simulink model "dr_screening_workflow"  (R2026a)
settings: Solver=FixedStepDiscrete  StopTime=sim_days*86400  FixedStep=fixed_step
values from neighbouring files (symbols this model uses):
  ai_time_s = 1.06    [run_workflow_sim.m]
  bandwidth_Mbps = 5    [run_workflow_sim.m]
  fixed_step = 5    [run_workflow_sim.m]
  image_MB = 0.35    [run_workflow_sim.m]
  images_per_patient = 2    [run_workflow_sim.m]
  n_ai_workers = 2    [run_workflow_sim.m]
  n_cameras = 6    [run_workflow_sim.m]
  n_reviewers = base_nr    (= 2)    [run_workflow_sim.m]
  patients_per_day = annual_volume/365    (= 273.97260274)    [run_workflow_sim.m]
  referral_frac = 0.30    (= 0.3)    [run_workflow_sim.m]
  review_time_s = 120    [run_workflow_sim.m]
  Tdrain = 60    [run_workflow_sim.m]
undefined symbols (not defined in the file or in its folder): DiscIntNeverNeededParam
settings Model: Creator=giridharansrinivasannaidu  LastModifiedBy=giridharansrinivasannaidu

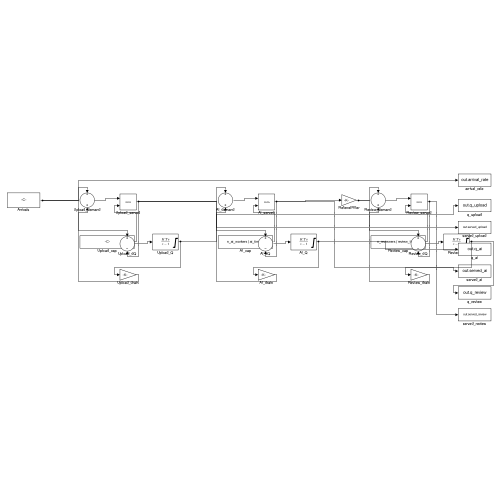
[thumbnail: Simulink's stored preview of the top-level diagram]
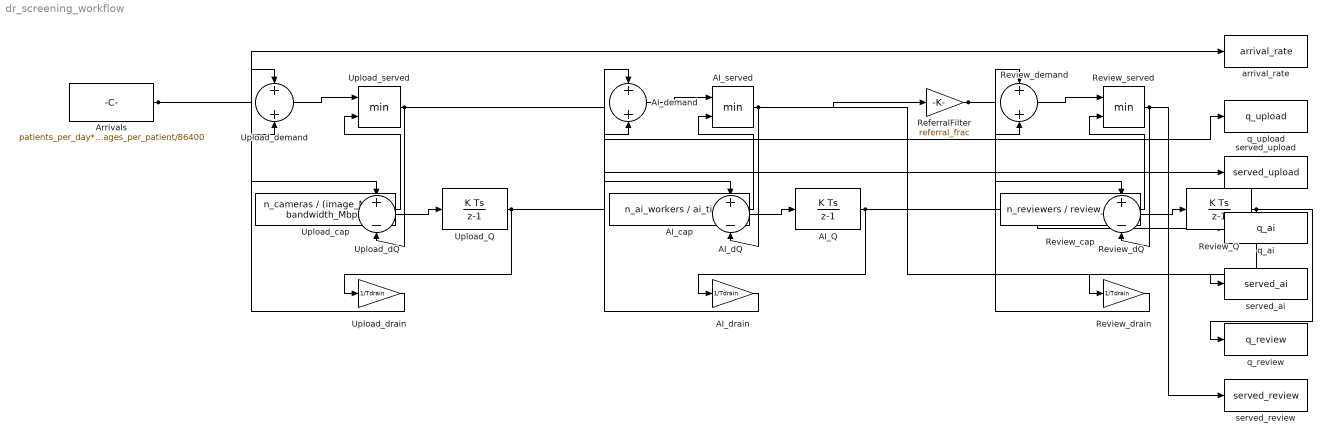
== system dr_screening_workflow ==
  AI_Q : DiscreteIntegrator  gainval=1  SampleTime=fixed_step  LimitOutput=on  LowerSaturationLimit=0  ICPrevOutput=DiscIntNeverNeededParam  ICPrevScaledInput=DiscIntNeverNeededParam
  AI_cap : Constant  Value=n_ai_workers / ai_time_s
  AI_dQ : Sum  Inputs=+-
  AI_demand : Sum
  AI_drain : Gain  Gain=1/Tdrain
  AI_served : MinMax  Inputs=2
  Arrivals : Constant  Value=patients_per_day*images_per_patient/86400
  ReferralFilter : Gain  Gain=referral_frac
  Review_Q : DiscreteIntegrator  gainval=1  SampleTime=fixed_step  LimitOutput=on  LowerSaturationLimit=0  ICPrevOutput=DiscIntNeverNeededParam  ICPrevScaledInput=DiscIntNeverNeededParam
  Review_cap : Constant  Value=n_reviewers / review_time_s
  Review_dQ : Sum  Inputs=+-
  Review_demand : Sum
  Review_drain : Gain  Gain=1/Tdrain
  Review_served : MinMax  Inputs=2
  Upload_Q : DiscreteIntegrator  gainval=1  SampleTime=fixed_step  LimitOutput=on  LowerSaturationLimit=0  ICPrevOutput=DiscIntNeverNeededParam  ICPrevScaledInput=DiscIntNeverNeededParam
  Upload_cap : Constant  Value=n_cameras / (image_MB*8 / bandwidth_Mbps)
  Upload_dQ : Sum  Inputs=+-
  Upload_demand : Sum
  Upload_drain : Gain  Gain=1/Tdrain
  Upload_served : MinMax  Inputs=2
  arrival_rate : ToWorkspace  VariableName=arrival_rate  SaveFormat=Timeseries  SampleTime=-1
      settings: Decimation=log_decim
  q_ai : ToWorkspace  VariableName=q_ai  SaveFormat=Timeseries  SampleTime=-1
      settings: Decimation=log_decim
  q_review : ToWorkspace  VariableName=q_review  SaveFormat=Timeseries  SampleTime=-1
      settings: Decimation=log_decim
  q_upload : ToWorkspace  VariableName=q_upload  SaveFormat=Timeseries  SampleTime=-1
      settings: Decimation=log_decim
  served_ai : ToWorkspace  VariableName=served_ai  SaveFormat=Timeseries  SampleTime=-1
      settings: Decimation=log_decim
  served_review : ToWorkspace  VariableName=served_review  SaveFormat=Timeseries  SampleTime=-1
      settings: Decimation=log_decim
  served_upload : ToWorkspace  VariableName=served_upload  SaveFormat=Timeseries  SampleTime=-1
      settings: Decimation=log_decim
  wires:
  Upload_demand/1 -> Upload_served/1
  Upload_cap/1 -> Upload_served/2
  Upload_served/1 -> Upload_dQ/2, AI_demand/1, AI_dQ/1, served_upload/1
  Upload_dQ/1 -> Upload_Q/1
  Upload_Q/1 -> Upload_drain/1, q_upload/1
  Upload_drain/1 -> Upload_demand/2
  AI_demand/1 -> AI_served/1
  AI_cap/1 -> AI_served/2
  AI_served/1 -> AI_dQ/2, ReferralFilter/1, served_ai/1
  AI_dQ/1 -> AI_Q/1
  AI_Q/1 -> AI_drain/1, q_ai/1
  AI_drain/1 -> AI_demand/2
  Review_demand/1 -> Review_served/1
  Review_cap/1 -> Review_served/2
  Review_served/1 -> Review_dQ/2, served_review/1
  Review_dQ/1 -> Review_Q/1
  Review_Q/1 -> Review_drain/1, q_review/1
  Review_drain/1 -> Review_demand/2
  Arrivals/1 -> Upload_demand/1, Upload_dQ/1, arrival_rate/1
  ReferralFilter/1 -> Review_demand/1, Review_dQ/1
